simulink model "orbitPropagator"  (R2020b)
settings: Solver=VariableStepAuto  StartTime=0.0  StopTime=10.0  RelTol=1e-3
values from neighbouring files (symbols this model uses):
  a = 6903    [constants.m]
  argp = 0    [constants.m]
  ecc = 0.003621614    [constants.m]
  incl = 1.701624178    [constants.m]
  RAAN = 3.96286888    [constants.m]
undefined symbols (not defined in the file or in its folder): magnitude
libraries: mspsensorlib x1
settings Model: Creator=ria_u  LastModifiedBy=khang

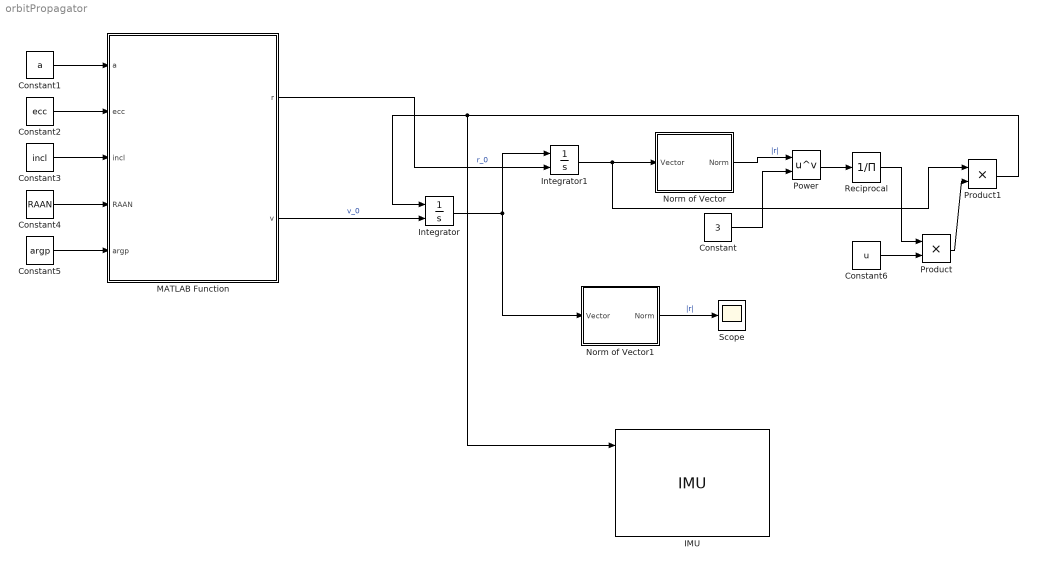
== system orbitPropagator ==
  Constant : Constant  Value=3
  Constant1 : Constant  Value=a
  Constant2 : Constant  Value=ecc
  Constant3 : Constant  Value=incl
  Constant4 : Constant  Value=RAAN
  Constant5 : Constant  Value=argp
  Constant6 : Constant  Value=u
  IMU : mspsensorlib/IMU  DispRefFrame=NED  Temperature=25  MagneticFieldNED=[ 27.5550, -2.4169, -16.0849 ]  MagneticFieldENU=[ -2.4169, 27.5550, 16.0849 ]  SeedDouble=67  SimulateUsing=Interpreted execution  AccelParamsMeasurementRange=Inf  AccelParamsResolution=0  AccelParamsConstantBias=[ 0, 0, 0 ]  AccelParamsAxesMisalignment=[ 0, 0, 0 ]  AccelParamsNoiseDensity=[ 0, 0, 0 ]  AccelParamsBiasInstability=[ 0, 0, 0 ]  AccelParamsRandomWalk=[ 0, 0, 0 ]  AccelParamsTemperatureBias=[ 0, 0, 0 ]  AccelParamsTemperatureScaleFactor=[ 0, 0, 0 ]  GyroParamsMeasurementRange=Inf  GyroParamsResolution=0  GyroParamsConstantBias=[ 0, 0, 0 ]  GyroParamsAxesMisalignment=[ 0, 0, 0 ]  GyroParamsAccelerationBias=[ 0, 0, 0 ]  GyroParamsNoiseDensity=[ 0, 0, 0 ]  GyroParamsBiasInstability=[ 0, 0, 0 ]  GyroParamsRandomWalk=[ 0, 0, 0 ]  GyroParamsTemperatureBias=[ 0, 0, 0 ]  GyroParamsTemperatureScaleFactor=[ 0, 0, 0 ]  MagParamsMeasurementRange=Inf  MagParamsResolution=0  MagParamsConstantBias=[ 0, 0, 0 ]  MagParamsAxesMisalignment=[ 0, 0, 0 ]  MagParamsNoiseDensity=[ 0, 0, 0 ]  MagParamsBiasInstability=[ 0, 0, 0 ]  MagParamsRandomWalk=[ 0, 0, 0 ]  MagParamsTemperatureBias=[ 0, 0, 0 ]  MagParamsTemperatureScaleFactor=[ 0, 0, 0 ]
      settings: SourceProductBaseCode=TF,NV
  Integrator : Integrator  InitialConditionSource=external
  Integrator1 : Integrator  InitialConditionSource=external
  MATLAB Function : MATLAB Function  TreatAsAtomicUnit=on
  Norm of Vector : Subsystem
  Norm of Vector1 : Subsystem
  Power : Math  Operator=pow  SaturateOnIntegerOverflow=on
  Product : Product
  Product1 : Product
  Reciprocal : Product  Inputs=/
  Scope : Scope
  wires:
  Constant3/1 -> MATLAB Function/3(incl)
  Constant4/1 -> MATLAB Function/4(RAAN)
  Constant2/1 -> MATLAB Function/2(ecc)
  Constant1/1 -> MATLAB Function/1(a)
  Constant5/1 -> MATLAB Function/5(argp)
  MATLAB Function/2(v) -> Integrator/2  "v_0"
  MATLAB Function/1(r) -> Integrator1/2  "r_0"
  Integrator1/1 -> Product1/1, Norm of Vector/1(Vector)
  Norm of Vector/1(Norm) -> Power/1  "|r|"
  Constant/1 -> Power/2
  Power/1 -> Reciprocal/1
  Reciprocal/1 -> Product/1
  Constant6/1 -> Product/2
  Product/1 -> Product1/2
  Product1/1 -> IMU/1, Integrator/1
  Integrator/1 -> Norm of Vector1/1(Vector), Integrator1/1
  Norm of Vector1/1(Norm) -> Scope/1  "|r|"

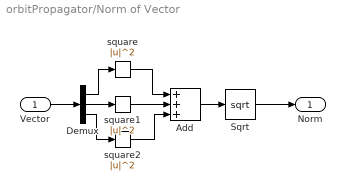
== system orbitPropagator/Norm of Vector ==
  Vector : Inport
  Add : Sum  Inputs=+++
  Demux : Demux  Outputs=3
  Sqrt : Sqrt  SaturateOnIntegerOverflow=on
  square : Math  Operator=magnitude^2  SaturateOnIntegerOverflow=on
  square1 : Math  Operator=magnitude^2  SaturateOnIntegerOverflow=on
  square2 : Math  Operator=magnitude^2  SaturateOnIntegerOverflow=on
  Norm : Outport
  wires:
  square2/1 -> Add/3
  Vector/1 -> Demux/1
  Sqrt/1 -> Norm/1
  Add/1 -> Sqrt/1
  Demux/3 -> square2/1
  square1/1 -> Add/2
  Demux/2 -> square1/1
  Demux/1 -> square/1
  square/1 -> Add/1

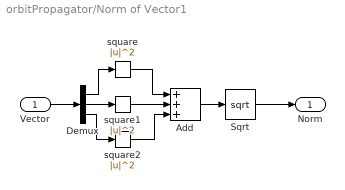
== system orbitPropagator/Norm of Vector1 ==
  Vector : Inport
  Add : Sum  Inputs=+++
  Demux : Demux  Outputs=3
  Sqrt : Sqrt  SaturateOnIntegerOverflow=on
  square : Math  Operator=magnitude^2  SaturateOnIntegerOverflow=on
  square1 : Math  Operator=magnitude^2  SaturateOnIntegerOverflow=on
  square2 : Math  Operator=magnitude^2  SaturateOnIntegerOverflow=on
  Norm : Outport
  wires:
  square2/1 -> Add/3
  Vector/1 -> Demux/1
  Sqrt/1 -> Norm/1
  Add/1 -> Sqrt/1
  Demux/3 -> square2/1
  square1/1 -> Add/2
  Demux/2 -> square1/1
  Demux/1 -> square/1
  square/1 -> Add/1

== matlab function orbitPropagator/MATLAB Function ==
  data: a input; r output; ecc input; incl input; RAAN input; argp input; v output
function [r, v] = init_conditions(a, ecc, incl, RAAN, argp)

    G = 6.6743e-20;      % Universal gravitational constant
    ME = 5.9724e24;      % Mass of Earth
    u = G*ME;            % Gravitational parameter of Earth
    
    C3w = [cos(argp), sin(argp), 0; -1*sin(argp), cos(argp), 0; 0, 0, 1]; 
    C1i = [1, 0, 0; 0, cos(incl), sin(incl); 0, -1*sin(incl), cos(incl)];
    C3O = [cos(RAAN), sin(RAAN), 0; -1*sin(RAAN), cos(RAAN), 0; 0, 0, 1];
    Cgp = (C3w*C1i*C3O)';    % Orbit to Earth rotation matrix
    
%     M = sqrt(u/a^3)*(t-t0);     % Mean anomaly
%     E = M;                      % First guess for Newton's Method
%     nmax = 15;                  % Max number of iterations desired
%     err = 1;                    % Initialize error value
%     n = 0;                      % Initialize iteration counter
%     
%     while (err>=1e-5 && n<=nmax)                      % Continues if the error is high and max # of loops have not occured
%         y = E - (E - (e*sin(E)) - M)/(1 - e*cos(E)); % Apply Newton's method
%         err = abs(E-y);                              % Calculate error
%         E = y;                                       % Replace eccentric anomaly with new value
%         n = n + 1;                                   % Update counter
%     end                                              % E is now the approximate eccentric anomaly
    
%    theta = 2*atan(sqrt((1+e)/(1-e))*tan(E/2));      % Calculates true anomaly

    theta = 0;
    R = (a*(1-ecc^2))/(1+ecc*cos(theta));                % Radial distance
    rp = [R*cos(theta);R*sin(theta);0];              % Position in perifocal frame
    vp = [-1*sin(theta);cos(theta)+ecc;0]*sqrt(u/(a*(1-ecc^2)));    % Velocity in perifocal frame
    
    r = Cgp*rp;       % Position in ECI
    v = Cgp*vp;       % Velocity in ECI
end
